simulink model "SecRwLtStBkReclnTrgtPosSelc"  (R2018b)
settings: Solver=FixedStepDiscrete  StartTime=0.0  StopTime=10.0  FixedStep=0.01  RelTol=1e-3
undefined symbols (not defined in the file): KeSMSw4SAcsMd21SecRwLtStBkReclnUpwdDnwdPos_Val, KeSMSw4SAcsMd21SecRwLtStBkReclnUpwdDnwdPosMax_Val, KeSMSw4SAcsMd21SecRwLtStBkReclnUpwdDnwdPosMin_Val, KeSMSw4SAcsMd22SecRwLtStBkReclnUpwdDnwdPos1_Val, KeSMSw4SAcsMd22SecRwLtStBkReclnUpwdDnwdPos1Max_Val, KeSMSw4SAcsMd22SecRwLtStBkReclnUpwdDnwdPos1Min_Val, KeSMSw4SAcsMd22SecRwLtStBkReclnUpwdDnwdPos2_Val, KeSMSw4SAcsMd22SecRwLtStBkReclnUpwdDnwdPos2Max_Val, KeSMSw4SAcsMd22SecRwLtStBkReclnUpwdDnwdPos2Min_Val, KeSMSw4SAcsMd25SecRwLtStBkReclnUpwdDnwdPos_Val, KeSMSw4SAcsMd25SecRwLtStBkReclnUpwdDnwdPosMax_Val, KeSMSw4SAcsMd25SecRwLtStBkReclnUpwdDnwdPosMin_Val, KeSMSw4SAcsMd26SecRwLtStBkReclnUpwdDnwdPos_Val, KeSMSw4SAcsMd26SecRwLtStBkReclnUpwdDnwdPosMax_Val, KeSMSw4SAcsMd26SecRwLtStBkReclnUpwdDnwdPosMin_Val, KeSMSw4sLyingMDSecRwLtStBkReclnUpwdDnwdPos_Val, KeSMSw4sLyingMDSecRwLtStBkReclnUpwdDnwdPosMax_Val, KeSMSw4sLyingMDSecRwLtStBkReclnUpwdDnwdPosMin_Val, KeSMSw4sRecoveryMDSecRwLtStBkReclnUpwdDnwdPos_Val, KeSMSw4sRecoveryMDSecRwLtStBkReclnUpwdDnwdPosMax_Val, KeSMSw4sRecoveryMDSecRwLtStBkReclnUpwdDnwdPosMin_Val, KeSMSw4sVIPMDSecRwLtStBkReclnUpwdDnwdPos_Val, KeSMSw4sVIPMDSecRwLtStBkReclnUpwdDnwdPosMax_Val, KeSMSw4sVIPMDSecRwLtStBkReclnUpwdDnwdPosMin_Val, KeSMSw6sAcsEntrySecRwLtStBkReclnUpwdDnwd1Pos_Val, KeSMSw6sAcsEntrySecRwLtStBkReclnUpwdDnwdPos1Max_Val, KeSMSw6sAcsEntrySecRwLtStBkReclnUpwdDnwdPos1Min_Val, KeSMSw6sAcsEntrySecRwLtStBkReclnUpwdDnwdPos_Val, KeSMSw6sAcsEntrySecRwLtStBkReclnUpwdDnwdPosMax_Val, KeSMSw6sAcsEntrySecRwLtStBkReclnUpwdDnwdPosMin_Val, KeSMSw6sAcsExtSecRwLtStBkReclnUpwdDnwdPos_Val, KeSMSw6sAcsExtSecRwLtStBkReclnUpwdDnwdPosMax_Val, KeSMSw6sAcsExtSecRwLtStBkReclnUpwdDnwdPosMin_Val, KeSMSw6sRecoveryMdSecRwLtStBkReclnUpwdDnwdPos_Val, KeSMSw6sRecoveryMdSecRwLtStBkReclnUpwdDnwdPosMax_Val, KeSMSw6sRecoveryMdSecRwLtStBkReclnUpwdDnwdPosMin_Val, KeSMSw6sVIPSecRwLtStBkReclnUpwdDnwdPos_Val, KeSMSw6sVIPSecRwLtStBkReclnUpwdDnwdPosMax_Val, KeSMSw6sVIPSecRwLtStBkReclnUpwdDnwdPosMin_Val, KeSMSwAcsEntrySecRwLtStBkReclnUpwdDnwdPos1_Val, KeSMSwAcsEntrySecRwLtStBkReclnUpwdDnwdPos1Max_Val, KeSMSwAcsEntrySecRwLtStBkReclnUpwdDnwdPos1Min_Val, KeSMSwAcsEntrySecRwLtStBkReclnUpwdDnwdPos_Val, KeSMSwAcsEntrySecRwLtStBkReclnUpwdDnwdPosMax_Val, KeSMSwAcsEntrySecRwLtStBkReclnUpwdDnwdPosMin_Val, KeSMSwAcsExtSecRwLtStBkReclnUpwdDnwdPos_Val, KeSMSwAcsExtSecRwLtStBkReclnUpwdDnwdPosMax_Val, KeSMSwAcsExtSecRwLtStBkReclnUpwdDnwdPosMin_Val, KeSMSwAcsMd32SecRwLtStBkReclnUpwdDnwdPos1_Val, KeSMSwAcsMd32SecRwLtStBkReclnUpwdDnwdPos1Max_Val, KeSMSwAcsMd32SecRwLtStBkReclnUpwdDnwdPos1Min_Val, KeSMSwAcsMd32SecRwLtStBkReclnUpwdDnwdPos_Val, KeSMSwAcsMd32SecRwLtStBkReclnUpwdDnwdPosMax_Val, KeSMSwAcsMd32SecRwLtStBkReclnUpwdDnwdPosMin_Val, KeSMSwAcsMd8SecRwLtStBkReclnUpwdDnwdPos_Val, KeSMSwAcsMd8SecRwLtStBkReclnUpwdDnwdPosMax_Val, KeSMSwAcsMd8SecRwLtStBkReclnUpwdDnwdPosMin_Val, KeSMSwRecoveryMdSecRwLtStBkReclnUpwdDnwdPos_Val, KeSMSwRecoveryMdSecRwLtStBkReclnUpwdDnwdPosMax_Val, KeSMSwRecoveryMdSecRwLtStBkReclnUpwdDnwdPosMin_Val ... (+3)
libraries: TrgtPosSelcLib x13, StIsPosChkLib x1, simulink x1
(part 1 of 2)
settings Model: Creator=sn2xws  LastModifiedBy=sn2xws
settings Model: ModifiedHistory=|
  | 2023.8.1 V2.0.0 CR421790 增加模式21-26
  | 2023.11.7 V2.3.0 bug 554442 md22 标定分为两套
  | 2024.5.7 557 eze模式变更
  | 2024.7.8 V3.0.1 557模式流程V1.9
  | 2024.8.17 V3.0.2 MD1靠背阶段1，2的选择逻辑变更
  | 2024.8.20 V3.0.3 Md32 目标位置改用Cush位置选择
settings DataIOCC: SaveFormat=StructureWithTime
settings OptimizationCC: DefaultParameterBehavior=Inlined  EnhancedBackFolding=on  PassReuseOutputArgsAs=Individual arguments  ZeroExternalMemoryAtStartup=off  ZeroInternalMemoryAtStartup=off  OptimizeBlockOrder=speed  DifferentSizesBufferReuse=on  OptimizationCustomize=off
settings DebuggingCC: ParameterTunabilityLossMsg=error
settings SFSimCC: MATLABDynamicMemAlloc=off
settings RTWCC: SystemTargetFile=autosar.tlc  GenCodeOnly=on  TemplateMakefile=ert_default_tmf  Description=AUTOSAR  GenerateReport=on  IncludeHyperlinkInReport=on  LaunchReport=on  GenerateTraceInfo=on  GenerateTraceReport=on  GenerateTraceReportSl=on  GenerateTraceReportSf=on  GenerateTraceReportEml=on  GenerateCodeMetricsReport=on
settings CodeAppCC: ForceParamTrailComments=on  IgnoreCustomStorageClasses=off  OperatorAnnotations=on  SimulinkDataObjDesc=on  SFDataObjDesc=on  InsertBlockDesc=on
settings STFCustomTargetCC: TargetLangStandard=C99 (ISO)  MultiwordLength=256  ParMdlRefBuildCompliant=on  CompOptLevelCompliant=on  IncludeMdlTerminateFcn=off  CombineOutputUpdateFcns=on  SuppressErrorStatus=on  ERTCustomFileBanners=on  SupportNonFinite=off  SupportComplex=off  SupportContinuousTime=off  SupportNonInlinedSFcns=off  RemoveResetFunc=on  MATLABClassNameForMDSCustomization=Simulink.SoftwareTarget.ERTCustomization  AutosarCompliant=on  UseToolchainInfoCompliant=on  LookupTableObjectStructAxisOrder=2,1,3,4,...  LUTObjectStructOrderEvenSpacing=Size,Table,Breakpoints  SystemTargetFile=autosar.tlc
settings ERTTargetCC: TargetLangStandard=C99 (ISO)  ConcurrentExecutionCompliant=off  IncludeMdlTerminateFcn=off  SuppressErrorStatus=on  SupportNonFinite=off  SupportComplex=off  ModelStepFunctionPrototypeControlCompliant=off  CPPClassGenCompliant=off  AutosarCompliant=on  LookupTableObjectStructAxisOrder=2,1,3,4,...  LUTObjectStructOrderEvenSpacing=Size,Table,Breakpoints  InlinedParameterPlacement=NonHierarchical  ERTCustomFileTemplate=example_file_process.tlc  ERTFilePackagingFormat=Compact

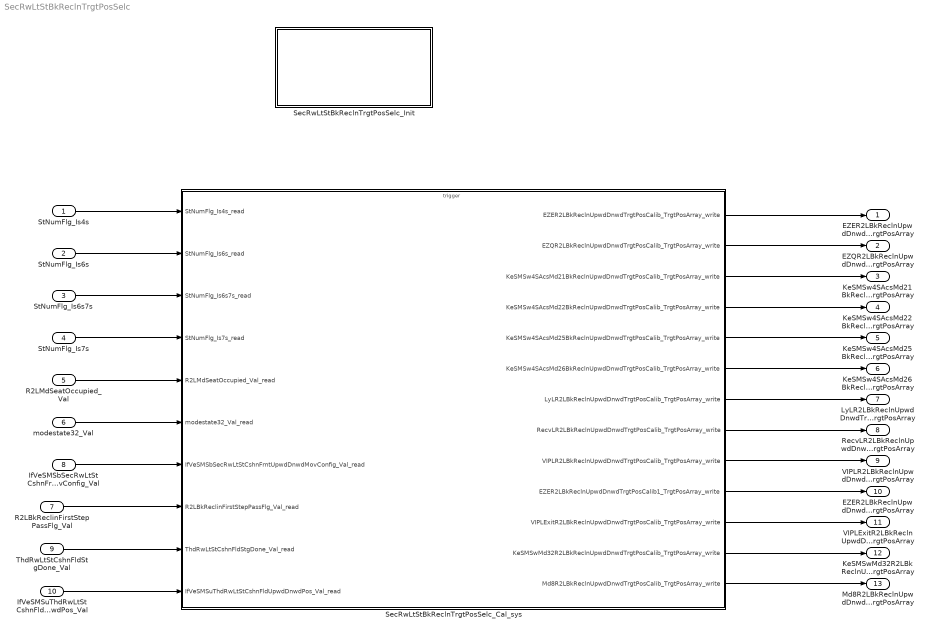
== system SecRwLtStBkReclnTrgtPosSelc ==
  StNumFlg_Is4s : Inport  OutDataTypeStr=boolean  PortDimensions=1
  StNumFlg_Is6s : Inport  Port=2  OutDataTypeStr=boolean  PortDimensions=1
  StNumFlg_Is6s7s : Inport  Port=3  OutDataTypeStr=boolean  PortDimensions=1
  StNumFlg_Is7s : Inport  Port=4  OutDataTypeStr=boolean  PortDimensions=1
  R2LMdSeatOccupied_Val : Inport  Port=5  OutDataTypeStr=boolean  PortDimensions=1
  modestate32_Val : Inport  Port=6  OutDataTypeStr=uint32  PortDimensions=1
  R2LBkReclinFirstStepPassFlg_Val : Inport  Port=7  OutDataTypeStr=boolean  PortDimensions=1
  IfVeSMSbSecRwLtStCshnFrntUpwdDnwdMovConfig_Val : Inport  Port=8  OutDataTypeStr=boolean  PortDimensions=1
  ThdRwLtStCshnFldStgDone_Val : Inport  Port=9  OutDataTypeStr=boolean  PortDimensions=1
  IfVeSMSuThdRwLtStCshnFldUpwdDnwdPos_Val : Inport  Port=10  OutDataTypeStr=uint16  PortDimensions=1
  SecRwLtStBkReclnTrgtPosSelc_Cal_sys : Subsystem
  SecRwLtStBkReclnTrgtPosSelc_Init : Subsystem
  EZER2LBkReclnUpwdDnwdTrgtPosCalib_TrgtPosArray : Outport  Description=|  OutDataTypeStr=uint16  PortDimensions=3
      | 0:Pos
      | 1:Max
      | 2:Min
  EZQR2LBkReclnUpwdDnwdTrgtPosCalib_TrgtPosArray : Outport  Description=|  Port=2  OutDataTypeStr=uint16  PortDimensions=3
      | 0:Pos
      | 1:Max
      | 2:Min
  KeSMSw4SAcsMd21BkReclnUpwdDnwdTrgtPosCalib_TrgtPosArray : Outport  Description=|  Port=3  OutDataTypeStr=uint16  PortDimensions=3
      | 0:Pos
      | 1:Max
      | 2:Min
  KeSMSw4SAcsMd22BkReclnUpwdDnwdTrgtPosCalib_TrgtPosArray : Outport  Description=|  Port=4  OutDataTypeStr=uint16  PortDimensions=3
      | 0:Pos
      | 1:Max
      | 2:Min
  KeSMSw4SAcsMd25BkReclnUpwdDnwdTrgtPosCalib_TrgtPosArray : Outport  Description=|  Port=5  OutDataTypeStr=uint16  PortDimensions=3
      | 0:Pos
      | 1:Max
      | 2:Min
  KeSMSw4SAcsMd26BkReclnUpwdDnwdTrgtPosCalib_TrgtPosArray : Outport  Description=|  Port=6  OutDataTypeStr=uint16  PortDimensions=3
      | 0:Pos
      | 1:Max
      | 2:Min
  LyLR2LBkReclnUpwdDnwdTrgtPosCalib_TrgtPosArray : Outport  Description=|  Port=7  OutDataTypeStr=uint16  PortDimensions=3
      | 0:Pos
      | 1:Max
      | 2:Min
  RecvLR2LBkReclnUpwdDnwdTrgtPosCalib_TrgtPosArray : Outport  Description=|  Port=8  OutDataTypeStr=uint16  PortDimensions=3
      | 0:Pos
      | 1:Max
      | 2:Min
  VIPLR2LBkReclnUpwdDnwdTrgtPosCalib_TrgtPosArray : Outport  Description=|  Port=9  OutDataTypeStr=uint16  PortDimensions=3
      | 0:Pos
      | 1:Max
      | 2:Min
  EZER2LBkReclnUpwdDnwdTrgtPosCalib1_TrgtPosArray : Outport  Description=|  Port=10  OutDataTypeStr=uint16  PortDimensions=3
      | 0:Pos
      | 1:Max
      | 2:Min
  VIPLExitR2LBkReclnUpwdDnwdTrgtPosCalib_TrgtPosArray : Outport  Description=|  Port=11  OutDataTypeStr=uint16  PortDimensions=3
      | 0:Pos
      | 1:Max
      | 2:Min
  KeSMSwMd32R2LBkReclnUpwdDnwdTrgtPosCalib_TrgtPosArray : Outport  Description=|  Port=12  OutDataTypeStr=uint16  PortDimensions=3
      | 0:Pos
      | 1:Max
      | 2:Min
  Md8R2LBkReclnUpwdDnwdTrgtPosCalib_TrgtPosArray : Outport  Description=|  Port=13  OutDataTypeStr=uint16  PortDimensions=3
      | 0:Pos
      | 1:Max
      | 2:Min
  wires:
  StNumFlg_Is4s/1 -> SecRwLtStBkReclnTrgtPosSelc_Cal_sys/1(StNumFlg_Is4s_read)
  StNumFlg_Is6s/1 -> SecRwLtStBkReclnTrgtPosSelc_Cal_sys/2(StNumFlg_Is6s_read)
  StNumFlg_Is6s7s/1 -> SecRwLtStBkReclnTrgtPosSelc_Cal_sys/3(StNumFlg_Is6s7s_read)
  StNumFlg_Is7s/1 -> SecRwLtStBkReclnTrgtPosSelc_Cal_sys/4(StNumFlg_Is7s_read)
  SecRwLtStBkReclnTrgtPosSelc_Cal_sys/1(EZER2LBkReclnUpwdDnwdTrgtPosCalib_TrgtPosArray_write) -> EZER2LBkReclnUpwdDnwdTrgtPosCalib_TrgtPosArray/1
  SecRwLtStBkReclnTrgtPosSelc_Cal_sys/2(EZQR2LBkReclnUpwdDnwdTrgtPosCalib_TrgtPosArray_write) -> EZQR2LBkReclnUpwdDnwdTrgtPosCalib_TrgtPosArray/1
  SecRwLtStBkReclnTrgtPosSelc_Cal_sys/3(KeSMSw4SAcsMd21BkReclnUpwdDnwdTrgtPosCalib_TrgtPosArray_write) -> KeSMSw4SAcsMd21BkReclnUpwdDnwdTrgtPosCalib_TrgtPosArray/1
  SecRwLtStBkReclnTrgtPosSelc_Cal_sys/4(KeSMSw4SAcsMd22BkReclnUpwdDnwdTrgtPosCalib_TrgtPosArray_write) -> KeSMSw4SAcsMd22BkReclnUpwdDnwdTrgtPosCalib_TrgtPosArray/1
  SecRwLtStBkReclnTrgtPosSelc_Cal_sys/5(KeSMSw4SAcsMd25BkReclnUpwdDnwdTrgtPosCalib_TrgtPosArray_write) -> KeSMSw4SAcsMd25BkReclnUpwdDnwdTrgtPosCalib_TrgtPosArray/1
  SecRwLtStBkReclnTrgtPosSelc_Cal_sys/6(KeSMSw4SAcsMd26BkReclnUpwdDnwdTrgtPosCalib_TrgtPosArray_write) -> KeSMSw4SAcsMd26BkReclnUpwdDnwdTrgtPosCalib_TrgtPosArray/1
  SecRwLtStBkReclnTrgtPosSelc_Cal_sys/7(LyLR2LBkReclnUpwdDnwdTrgtPosCalib_TrgtPosArray_write) -> LyLR2LBkReclnUpwdDnwdTrgtPosCalib_TrgtPosArray/1
  SecRwLtStBkReclnTrgtPosSelc_Cal_sys/8(RecvLR2LBkReclnUpwdDnwdTrgtPosCalib_TrgtPosArray_write) -> RecvLR2LBkReclnUpwdDnwdTrgtPosCalib_TrgtPosArray/1
  SecRwLtStBkReclnTrgtPosSelc_Cal_sys/9(VIPLR2LBkReclnUpwdDnwdTrgtPosCalib_TrgtPosArray_write) -> VIPLR2LBkReclnUpwdDnwdTrgtPosCalib_TrgtPosArray/1
  R2LMdSeatOccupied_Val/1 -> SecRwLtStBkReclnTrgtPosSelc_Cal_sys/5(R2LMdSeatOccupied_Val_read)
  SecRwLtStBkReclnTrgtPosSelc_Cal_sys/10(EZER2LBkReclnUpwdDnwdTrgtPosCalib1_TrgtPosArray_write) -> EZER2LBkReclnUpwdDnwdTrgtPosCalib1_TrgtPosArray/1
  modestate32_Val/1 -> SecRwLtStBkReclnTrgtPosSelc_Cal_sys/6(modestate32_Val_read)
  R2LBkReclinFirstStepPassFlg_Val/1 -> SecRwLtStBkReclnTrgtPosSelc_Cal_sys/8(R2LBkReclinFirstStepPassFlg_Val_read)
  IfVeSMSbSecRwLtStCshnFrntUpwdDnwdMovConfig_Val/1 -> SecRwLtStBkReclnTrgtPosSelc_Cal_sys/7(IfVeSMSbSecRwLtStCshnFrntUpwdDnwdMovConfig_Val_read)
  SecRwLtStBkReclnTrgtPosSelc_Cal_sys/11(VIPLExitR2LBkReclnUpwdDnwdTrgtPosCalib_TrgtPosArray_write) -> VIPLExitR2LBkReclnUpwdDnwdTrgtPosCalib_TrgtPosArray/1
  ThdRwLtStCshnFldStgDone_Val/1 -> SecRwLtStBkReclnTrgtPosSelc_Cal_sys/9(ThdRwLtStCshnFldStgDone_Val_read)
  SecRwLtStBkReclnTrgtPosSelc_Cal_sys/12(KeSMSwMd32R2LBkReclnUpwdDnwdTrgtPosCalib_TrgtPosArray_write) -> KeSMSwMd32R2LBkReclnUpwdDnwdTrgtPosCalib_TrgtPosArray/1
  SecRwLtStBkReclnTrgtPosSelc_Cal_sys/13(Md8R2LBkReclnUpwdDnwdTrgtPosCalib_TrgtPosArray_write) -> Md8R2LBkReclnUpwdDnwdTrgtPosCalib_TrgtPosArray/1
  IfVeSMSuThdRwLtStCshnFldUpwdDnwdPos_Val/1 -> SecRwLtStBkReclnTrgtPosSelc_Cal_sys/10(IfVeSMSuThdRwLtStCshnFldUpwdDnwdPos_Val_read)

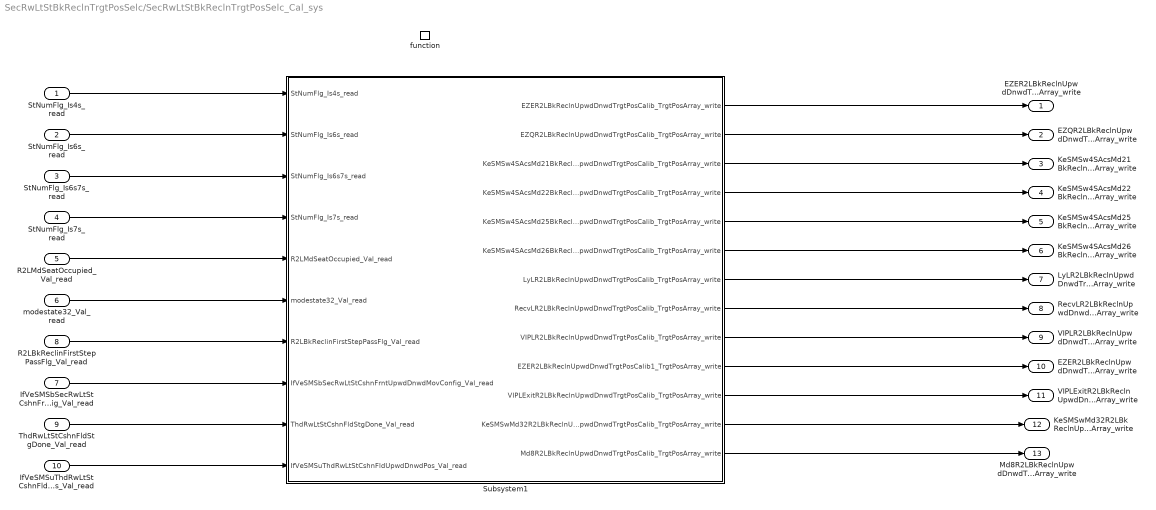
== system SecRwLtStBkReclnTrgtPosSelc/SecRwLtStBkReclnTrgtPosSelc_Cal_sys ==
  StNumFlg_Is4s_read : Inport
  StNumFlg_Is6s_read : Inport  Port=2
  StNumFlg_Is6s7s_read : Inport  Port=3
  StNumFlg_Is7s_read : Inport  Port=4
  R2LMdSeatOccupied_Val_read : Inport  Port=5
  modestate32_Val_read : Inport  Port=6
  IfVeSMSbSecRwLtStCshnFrntUpwdDnwdMovConfig_Val_read : Inport  Port=7
  R2LBkReclinFirstStepPassFlg_Val_read : Inport  Port=8
  ThdRwLtStCshnFldStgDone_Val_read : Inport  Port=9
  IfVeSMSuThdRwLtStCshnFldUpwdDnwdPos_Val_read : Inport  Port=10
  function : TriggerPort  TriggerType=function-call  IsSimulinkFunction=on  FunctionName=SecRwLtStBkReclnTrgtPosSelc_Cal  VariantControl=(inherit)
  Subsystem1 : Subsystem
  EZER2LBkReclnUpwdDnwdTrgtPosCalib_TrgtPosArray_write : Outport
      settings: EnsureOutportIsVirtual=on
  EZQR2LBkReclnUpwdDnwdTrgtPosCalib_TrgtPosArray_write : Outport  Port=2
      settings: EnsureOutportIsVirtual=on
  KeSMSw4SAcsMd21BkReclnUpwdDnwdTrgtPosCalib_TrgtPosArray_write : Outport  Port=3
      settings: EnsureOutportIsVirtual=on
  KeSMSw4SAcsMd22BkReclnUpwdDnwdTrgtPosCalib_TrgtPosArray_write : Outport  Port=4
      settings: EnsureOutportIsVirtual=on
  KeSMSw4SAcsMd25BkReclnUpwdDnwdTrgtPosCalib_TrgtPosArray_write : Outport  Port=5
      settings: EnsureOutportIsVirtual=on
  KeSMSw4SAcsMd26BkReclnUpwdDnwdTrgtPosCalib_TrgtPosArray_write : Outport  Port=6
      settings: EnsureOutportIsVirtual=on
  LyLR2LBkReclnUpwdDnwdTrgtPosCalib_TrgtPosArray_write : Outport  Port=7
      settings: EnsureOutportIsVirtual=on
  RecvLR2LBkReclnUpwdDnwdTrgtPosCalib_TrgtPosArray_write : Outport  Port=8
      settings: EnsureOutportIsVirtual=on
  VIPLR2LBkReclnUpwdDnwdTrgtPosCalib_TrgtPosArray_write : Outport  Port=9
      settings: EnsureOutportIsVirtual=on
  EZER2LBkReclnUpwdDnwdTrgtPosCalib1_TrgtPosArray_write : Outport  Port=10
      settings: EnsureOutportIsVirtual=on
  VIPLExitR2LBkReclnUpwdDnwdTrgtPosCalib_TrgtPosArray_write : Outport  Port=11
      settings: EnsureOutportIsVirtual=on
  KeSMSwMd32R2LBkReclnUpwdDnwdTrgtPosCalib_TrgtPosArray_write : Outport  Port=12
      settings: EnsureOutportIsVirtual=on
  Md8R2LBkReclnUpwdDnwdTrgtPosCalib_TrgtPosArray_write : Outport  Port=13
      settings: EnsureOutportIsVirtual=on
  wires:
  Subsystem1/6(KeSMSw4SAcsMd26BkReclnUpwdDnwdTrgtPosCalib_TrgtPosArray_write) -> KeSMSw4SAcsMd26BkReclnUpwdDnwdTrgtPosCalib_TrgtPosArray_write/1
  Subsystem1/7(LyLR2LBkReclnUpwdDnwdTrgtPosCalib_TrgtPosArray_write) -> LyLR2LBkReclnUpwdDnwdTrgtPosCalib_TrgtPosArray_write/1
  Subsystem1/8(RecvLR2LBkReclnUpwdDnwdTrgtPosCalib_TrgtPosArray_write) -> RecvLR2LBkReclnUpwdDnwdTrgtPosCalib_TrgtPosArray_write/1
  Subsystem1/4(KeSMSw4SAcsMd22BkReclnUpwdDnwdTrgtPosCalib_TrgtPosArray_write) -> KeSMSw4SAcsMd22BkReclnUpwdDnwdTrgtPosCalib_TrgtPosArray_write/1
  Subsystem1/5(KeSMSw4SAcsMd25BkReclnUpwdDnwdTrgtPosCalib_TrgtPosArray_write) -> KeSMSw4SAcsMd25BkReclnUpwdDnwdTrgtPosCalib_TrgtPosArray_write/1
  Subsystem1/9(VIPLR2LBkReclnUpwdDnwdTrgtPosCalib_TrgtPosArray_write) -> VIPLR2LBkReclnUpwdDnwdTrgtPosCalib_TrgtPosArray_write/1
  Subsystem1/1(EZER2LBkReclnUpwdDnwdTrgtPosCalib_TrgtPosArray_write) -> EZER2LBkReclnUpwdDnwdTrgtPosCalib_TrgtPosArray_write/1
  Subsystem1/2(EZQR2LBkReclnUpwdDnwdTrgtPosCalib_TrgtPosArray_write) -> EZQR2LBkReclnUpwdDnwdTrgtPosCalib_TrgtPosArray_write/1
  Subsystem1/3(KeSMSw4SAcsMd21BkReclnUpwdDnwdTrgtPosCalib_TrgtPosArray_write) -> KeSMSw4SAcsMd21BkReclnUpwdDnwdTrgtPosCalib_TrgtPosArray_write/1
  StNumFlg_Is4s_read/1 -> Subsystem1/1(StNumFlg_Is4s_read)
  StNumFlg_Is6s_read/1 -> Subsystem1/2(StNumFlg_Is6s_read)
  StNumFlg_Is6s7s_read/1 -> Subsystem1/3(StNumFlg_Is6s7s_read)
  StNumFlg_Is7s_read/1 -> Subsystem1/4(StNumFlg_Is7s_read)
  R2LMdSeatOccupied_Val_read/1 -> Subsystem1/5(R2LMdSeatOccupied_Val_read)
  Subsystem1/10(EZER2LBkReclnUpwdDnwdTrgtPosCalib1_TrgtPosArray_write) -> EZER2LBkReclnUpwdDnwdTrgtPosCalib1_TrgtPosArray_write/1
  modestate32_Val_read/1 -> Subsystem1/6(modestate32_Val_read)
  IfVeSMSbSecRwLtStCshnFrntUpwdDnwdMovConfig_Val_read/1 -> Subsystem1/8(IfVeSMSbSecRwLtStCshnFrntUpwdDnwdMovConfig_Val_read)
  Subsystem1/11(VIPLExitR2LBkReclnUpwdDnwdTrgtPosCalib_TrgtPosArray_write) -> VIPLExitR2LBkReclnUpwdDnwdTrgtPosCalib_TrgtPosArray_write/1
  Subsystem1/12(KeSMSwMd32R2LBkReclnUpwdDnwdTrgtPosCalib_TrgtPosArray_write) -> KeSMSwMd32R2LBkReclnUpwdDnwdTrgtPosCalib_TrgtPosArray_write/1
  Subsystem1/13(Md8R2LBkReclnUpwdDnwdTrgtPosCalib_TrgtPosArray_write) -> Md8R2LBkReclnUpwdDnwdTrgtPosCalib_TrgtPosArray_write/1
  R2LBkReclinFirstStepPassFlg_Val_read/1 -> Subsystem1/7(R2LBkReclinFirstStepPassFlg_Val_read)
  ThdRwLtStCshnFldStgDone_Val_read/1 -> Subsystem1/9(ThdRwLtStCshnFldStgDone_Val_read)
  IfVeSMSuThdRwLtStCshnFldUpwdDnwdPos_Val_read/1 -> Subsystem1/10(IfVeSMSuThdRwLtStCshnFldUpwdDnwdPos_Val_read)

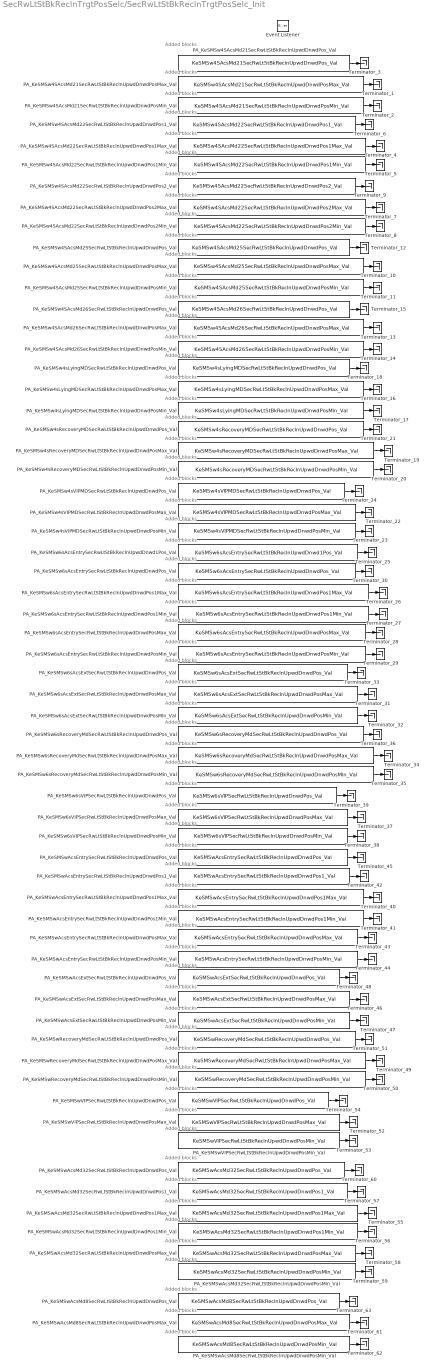
== system SecRwLtStBkReclnTrgtPosSelc/SecRwLtStBkReclnTrgtPosSelc_Init ==
  note: Added blocks
  note: Added blocks
  note: Added blocks
  note: Added blocks
  note: Added blocks
  note: Added blocks
  note: Added blocks
  note: Added blocks
  note: Added blocks
  note: Added blocks
  note: Added blocks
  note: Added blocks
  note: Added blocks
  note: Added blocks
  note: Added blocks
  note: Added blocks
  note: Added blocks
  note: Added blocks
  note: Added blocks
  note: Added blocks
  note: Added blocks
  note: Added blocks
  note: Added blocks
  note: Added blocks
  note: Added blocks
  note: Added blocks
  note: Added blocks
  note: Added blocks
  note: Added blocks
  note: Added blocks
  note: Added blocks
  note: Added blocks
  note: Added blocks
  note: Added blocks
  note: Added blocks
  note: Added blocks
  note: Added blocks
  note: Added blocks
  note: Added blocks
  note: Added blocks
  note: Added blocks
  note: Added blocks
  note: Added blocks
  note: Added blocks
  note: Added blocks
  note: Added blocks
  note: Added blocks
  note: Added blocks
  note: Added blocks
  note: Added blocks
  note: Added blocks
  note: Added blocks
  note: Added blocks
  note: Added blocks
  note: Added blocks
  note: Added blocks
  note: Added blocks
  note: Added blocks
  note: Added blocks
  note: Added blocks
  note: Added blocks
  note: Added blocks
  note: Added blocks
  Event Listener : EventListener  EventName=reset
  PA_KeSMSw4SAcsMd21SecRwLtStBkReclnUpwdDnwdPosMax_Val : Constant  Value=KeSMSw4SAcsMd21SecRwLtStBkReclnUpwdDnwdPosMax_Val
  PA_KeSMSw4SAcsMd21SecRwLtStBkReclnUpwdDnwdPosMin_Val : Constant  Value=KeSMSw4SAcsMd21SecRwLtStBkReclnUpwdDnwdPosMin_Val
  PA_KeSMSw4SAcsMd21SecRwLtStBkReclnUpwdDnwdPos_Val : Constant  Value=KeSMSw4SAcsMd21SecRwLtStBkReclnUpwdDnwdPos_Val
  PA_KeSMSw4SAcsMd22SecRwLtStBkReclnUpwdDnwdPos1Max_Val : Constant  Value=KeSMSw4SAcsMd22SecRwLtStBkReclnUpwdDnwdPos1Max_Val
  PA_KeSMSw4SAcsMd22SecRwLtStBkReclnUpwdDnwdPos1Min_Val : Constant  Value=KeSMSw4SAcsMd22SecRwLtStBkReclnUpwdDnwdPos1Min_Val
  PA_KeSMSw4SAcsMd22SecRwLtStBkReclnUpwdDnwdPos1_Val : Constant  Value=KeSMSw4SAcsMd22SecRwLtStBkReclnUpwdDnwdPos1_Val
  PA_KeSMSw4SAcsMd22SecRwLtStBkReclnUpwdDnwdPos2Max_Val : Constant  Value=KeSMSw4SAcsMd22SecRwLtStBkReclnUpwdDnwdPos2Max_Val
  PA_KeSMSw4SAcsMd22SecRwLtStBkReclnUpwdDnwdPos2Min_Val : Constant  Value=KeSMSw4SAcsMd22SecRwLtStBkReclnUpwdDnwdPos2Min_Val
  PA_KeSMSw4SAcsMd22SecRwLtStBkReclnUpwdDnwdPos2_Val : Constant  Value=KeSMSw4SAcsMd22SecRwLtStBkReclnUpwdDnwdPos2_Val
  PA_KeSMSw4SAcsMd25SecRwLtStBkReclnUpwdDnwdPosMax_Val : Constant  Value=KeSMSw4SAcsMd25SecRwLtStBkReclnUpwdDnwdPosMax_Val
  PA_KeSMSw4SAcsMd25SecRwLtStBkReclnUpwdDnwdPosMin_Val : Constant  Value=KeSMSw4SAcsMd25SecRwLtStBkReclnUpwdDnwdPosMin_Val
  PA_KeSMSw4SAcsMd25SecRwLtStBkReclnUpwdDnwdPos_Val : Constant  Value=KeSMSw4SAcsMd25SecRwLtStBkReclnUpwdDnwdPos_Val
  PA_KeSMSw4SAcsMd26SecRwLtStBkReclnUpwdDnwdPosMax_Val : Constant  Value=KeSMSw4SAcsMd26SecRwLtStBkReclnUpwdDnwdPosMax_Val
  PA_KeSMSw4SAcsMd26SecRwLtStBkReclnUpwdDnwdPosMin_Val : Constant  Value=KeSMSw4SAcsMd26SecRwLtStBkReclnUpwdDnwdPosMin_Val
  PA_KeSMSw4SAcsMd26SecRwLtStBkReclnUpwdDnwdPos_Val : Constant  Value=KeSMSw4SAcsMd26SecRwLtStBkReclnUpwdDnwdPos_Val
  PA_KeSMSw4sLyingMDSecRwLtStBkReclnUpwdDnwdPosMax_Val : Constant  Value=KeSMSw4sLyingMDSecRwLtStBkReclnUpwdDnwdPosMax_Val
  PA_KeSMSw4sLyingMDSecRwLtStBkReclnUpwdDnwdPosMin_Val : Constant  Value=KeSMSw4sLyingMDSecRwLtStBkReclnUpwdDnwdPosMin_Val
  PA_KeSMSw4sLyingMDSecRwLtStBkReclnUpwdDnwdPos_Val : Constant  Value=KeSMSw4sLyingMDSecRwLtStBkReclnUpwdDnwdPos_Val
  PA_KeSMSw4sRecoveryMDSecRwLtStBkReclnUpwdDnwdPosMax_Val : Constant  Value=KeSMSw4sRecoveryMDSecRwLtStBkReclnUpwdDnwdPosMax_Val
  PA_KeSMSw4sRecoveryMDSecRwLtStBkReclnUpwdDnwdPosMin_Val : Constant  Value=KeSMSw4sRecoveryMDSecRwLtStBkReclnUpwdDnwdPosMin_Val
  PA_KeSMSw4sRecoveryMDSecRwLtStBkReclnUpwdDnwdPos_Val : Constant  Value=KeSMSw4sRecoveryMDSecRwLtStBkReclnUpwdDnwdPos_Val
  PA_KeSMSw4sVIPMDSecRwLtStBkReclnUpwdDnwdPosMax_Val : Constant  Value=KeSMSw4sVIPMDSecRwLtStBkReclnUpwdDnwdPosMax_Val
  PA_KeSMSw4sVIPMDSecRwLtStBkReclnUpwdDnwdPosMin_Val : Constant  Value=KeSMSw4sVIPMDSecRwLtStBkReclnUpwdDnwdPosMin_Val
  PA_KeSMSw4sVIPMDSecRwLtStBkReclnUpwdDnwdPos_Val : Constant  Value=KeSMSw4sVIPMDSecRwLtStBkReclnUpwdDnwdPos_Val
  PA_KeSMSw6sAcsEntrySecRwLtStBkReclnUpwdDnwd1Pos_Val : Constant  Value=KeSMSw6sAcsEntrySecRwLtStBkReclnUpwdDnwd1Pos_Val
  PA_KeSMSw6sAcsEntrySecRwLtStBkReclnUpwdDnwdPos1Max_Val : Constant  Value=KeSMSw6sAcsEntrySecRwLtStBkReclnUpwdDnwdPos1Max_Val
  PA_KeSMSw6sAcsEntrySecRwLtStBkReclnUpwdDnwdPos1Min_Val : Constant  Value=KeSMSw6sAcsEntrySecRwLtStBkReclnUpwdDnwdPos1Min_Val
  PA_KeSMSw6sAcsEntrySecRwLtStBkReclnUpwdDnwdPosMax_Val : Constant  Value=KeSMSw6sAcsEntrySecRwLtStBkReclnUpwdDnwdPosMax_Val
  PA_KeSMSw6sAcsEntrySecRwLtStBkReclnUpwdDnwdPosMin_Val : Constant  Value=KeSMSw6sAcsEntrySecRwLtStBkReclnUpwdDnwdPosMin_Val
  PA_KeSMSw6sAcsEntrySecRwLtStBkReclnUpwdDnwdPos_Val : Constant  Value=KeSMSw6sAcsEntrySecRwLtStBkReclnUpwdDnwdPos_Val
  PA_KeSMSw6sAcsExtSecRwLtStBkReclnUpwdDnwdPosMax_Val : Constant  Value=KeSMSw6sAcsExtSecRwLtStBkReclnUpwdDnwdPosMax_Val
  PA_KeSMSw6sAcsExtSecRwLtStBkReclnUpwdDnwdPosMin_Val : Constant  Value=KeSMSw6sAcsExtSecRwLtStBkReclnUpwdDnwdPosMin_Val
  PA_KeSMSw6sAcsExtSecRwLtStBkReclnUpwdDnwdPos_Val : Constant  Value=KeSMSw6sAcsExtSecRwLtStBkReclnUpwdDnwdPos_Val
  PA_KeSMSw6sRecoveryMdSecRwLtStBkReclnUpwdDnwdPosMax_Val : Constant  Value=KeSMSw6sRecoveryMdSecRwLtStBkReclnUpwdDnwdPosMax_Val
  PA_KeSMSw6sRecoveryMdSecRwLtStBkReclnUpwdDnwdPosMin_Val : Constant  Value=KeSMSw6sRecoveryMdSecRwLtStBkReclnUpwdDnwdPosMin_Val
  PA_KeSMSw6sRecoveryMdSecRwLtStBkReclnUpwdDnwdPos_Val : Constant  Value=KeSMSw6sRecoveryMdSecRwLtStBkReclnUpwdDnwdPos_Val
  PA_KeSMSw6sVIPSecRwLtStBkReclnUpwdDnwdPosMax_Val : Constant  Value=KeSMSw6sVIPSecRwLtStBkReclnUpwdDnwdPosMax_Val
  PA_KeSMSw6sVIPSecRwLtStBkReclnUpwdDnwdPosMin_Val : Constant  Value=KeSMSw6sVIPSecRwLtStBkReclnUpwdDnwdPosMin_Val
  PA_KeSMSw6sVIPSecRwLtStBkReclnUpwdDnwdPos_Val : Constant  Value=KeSMSw6sVIPSecRwLtStBkReclnUpwdDnwdPos_Val
  PA_KeSMSwAcsEntrySecRwLtStBkReclnUpwdDnwdPos1Max_Val : Constant  Value=KeSMSwAcsEntrySecRwLtStBkReclnUpwdDnwdPos1Max_Val
  PA_KeSMSwAcsEntrySecRwLtStBkReclnUpwdDnwdPos1Min_Val : Constant  Value=KeSMSwAcsEntrySecRwLtStBkReclnUpwdDnwdPos1Min_Val
  PA_KeSMSwAcsEntrySecRwLtStBkReclnUpwdDnwdPos1_Val : Constant  Value=KeSMSwAcsEntrySecRwLtStBkReclnUpwdDnwdPos1_Val
  PA_KeSMSwAcsEntrySecRwLtStBkReclnUpwdDnwdPosMax_Val : Constant  Value=KeSMSwAcsEntrySecRwLtStBkReclnUpwdDnwdPosMax_Val
  PA_KeSMSwAcsEntrySecRwLtStBkReclnUpwdDnwdPosMin_Val : Constant  Value=KeSMSwAcsEntrySecRwLtStBkReclnUpwdDnwdPosMin_Val
  PA_KeSMSwAcsEntrySecRwLtStBkReclnUpwdDnwdPos_Val : Constant  Value=KeSMSwAcsEntrySecRwLtStBkReclnUpwdDnwdPos_Val
  PA_KeSMSwAcsExtSecRwLtStBkReclnUpwdDnwdPosMax_Val : Constant  Value=KeSMSwAcsExtSecRwLtStBkReclnUpwdDnwdPosMax_Val
  PA_KeSMSwAcsExtSecRwLtStBkReclnUpwdDnwdPosMin_Val : Constant  Value=KeSMSwAcsExtSecRwLtStBkReclnUpwdDnwdPosMin_Val
  PA_KeSMSwAcsExtSecRwLtStBkReclnUpwdDnwdPos_Val : Constant  Value=KeSMSwAcsExtSecRwLtStBkReclnUpwdDnwdPos_Val
  PA_KeSMSwAcsMd32SecRwLtStBkReclnUpwdDnwdPos1Max_Val : Constant  Value=KeSMSwAcsMd32SecRwLtStBkReclnUpwdDnwdPos1Max_Val
  PA_KeSMSwAcsMd32SecRwLtStBkReclnUpwdDnwdPos1Min_Val : Constant  Value=KeSMSwAcsMd32SecRwLtStBkReclnUpwdDnwdPos1Min_Val
  PA_KeSMSwAcsMd32SecRwLtStBkReclnUpwdDnwdPos1_Val : Constant  Value=KeSMSwAcsMd32SecRwLtStBkReclnUpwdDnwdPos1_Val
  PA_KeSMSwAcsMd32SecRwLtStBkReclnUpwdDnwdPosMax_Val : Constant  Value=KeSMSwAcsMd32SecRwLtStBkReclnUpwdDnwdPosMax_Val
  PA_KeSMSwAcsMd32SecRwLtStBkReclnUpwdDnwdPosMin_Val : Constant  Value=KeSMSwAcsMd32SecRwLtStBkReclnUpwdDnwdPosMin_Val
  PA_KeSMSwAcsMd32SecRwLtStBkReclnUpwdDnwdPos_Val : Constant  Value=KeSMSwAcsMd32SecRwLtStBkReclnUpwdDnwdPos_Val
  PA_KeSMSwAcsMd8SecRwLtStBkReclnUpwdDnwdPosMax_Val : Constant  Value=KeSMSwAcsMd8SecRwLtStBkReclnUpwdDnwdPosMax_Val
  PA_KeSMSwAcsMd8SecRwLtStBkReclnUpwdDnwdPosMin_Val : Constant  Value=KeSMSwAcsMd8SecRwLtStBkReclnUpwdDnwdPosMin_Val
  PA_KeSMSwAcsMd8SecRwLtStBkReclnUpwdDnwdPos_Val : Constant  Value=KeSMSwAcsMd8SecRwLtStBkReclnUpwdDnwdPos_Val
  PA_KeSMSwRecoveryMdSecRwLtStBkReclnUpwdDnwdPosMax_Val : Constant  Value=KeSMSwRecoveryMdSecRwLtStBkReclnUpwdDnwdPosMax_Val
  PA_KeSMSwRecoveryMdSecRwLtStBkReclnUpwdDnwdPosMin_Val : Constant  Value=KeSMSwRecoveryMdSecRwLtStBkReclnUpwdDnwdPosMin_Val
  PA_KeSMSwRecoveryMdSecRwLtStBkReclnUpwdDnwdPos_Val : Constant  Value=KeSMSwRecoveryMdSecRwLtStBkReclnUpwdDnwdPos_Val
  PA_KeSMSwVIPSecRwLtStBkReclnUpwdDnwdPosMax_Val : Constant  Value=KeSMSwVIPSecRwLtStBkReclnUpwdDnwdPosMax_Val
  PA_KeSMSwVIPSecRwLtStBkReclnUpwdDnwdPosMin_Val : Constant  Value=KeSMSwVIPSecRwLtStBkReclnUpwdDnwdPosMin_Val
  PA_KeSMSwVIPSecRwLtStBkReclnUpwdDnwdPos_Val : Constant  Value=KeSMSwVIPSecRwLtStBkReclnUpwdDnwdPos_Val
  Terminator_{1..63} (63 alike) : Terminator
  wires:
  PA_KeSMSw4SAcsMd21SecRwLtStBkReclnUpwdDnwdPosMax_Val/1 -> Terminator_1/1
  PA_KeSMSw4SAcsMd21SecRwLtStBkReclnUpwdDnwdPosMin_Val/1 -> Terminator_2/1
  PA_KeSMSw4SAcsMd21SecRwLtStBkReclnUpwdDnwdPos_Val/1 -> Terminator_3/1
  PA_KeSMSw4SAcsMd22SecRwLtStBkReclnUpwdDnwdPos1Max_Val/1 -> Terminator_4/1
  PA_KeSMSw4SAcsMd22SecRwLtStBkReclnUpwdDnwdPos1Min_Val/1 -> Terminator_5/1
  PA_KeSMSw4SAcsMd22SecRwLtStBkReclnUpwdDnwdPos1_Val/1 -> Terminator_6/1
  PA_KeSMSw4SAcsMd22SecRwLtStBkReclnUpwdDnwdPos2Max_Val/1 -> Terminator_7/1
  PA_KeSMSw4SAcsMd22SecRwLtStBkReclnUpwdDnwdPos2Min_Val/1 -> Terminator_8/1
  PA_KeSMSw4SAcsMd22SecRwLtStBkReclnUpwdDnwdPos2_Val/1 -> Terminator_9/1
  PA_KeSMSw4SAcsMd25SecRwLtStBkReclnUpwdDnwdPosMax_Val/1 -> Terminator_10/1
  PA_KeSMSw4SAcsMd25SecRwLtStBkReclnUpwdDnwdPosMin_Val/1 -> Terminator_11/1
  PA_KeSMSw4SAcsMd25SecRwLtStBkReclnUpwdDnwdPos_Val/1 -> Terminator_12/1
  PA_KeSMSw4SAcsMd26SecRwLtStBkReclnUpwdDnwdPosMax_Val/1 -> Terminator_13/1
  PA_KeSMSw4SAcsMd26SecRwLtStBkReclnUpwdDnwdPosMin_Val/1 -> Terminator_14/1
  PA_KeSMSw4SAcsMd26SecRwLtStBkReclnUpwdDnwdPos_Val/1 -> Terminator_15/1
  PA_KeSMSw4sLyingMDSecRwLtStBkReclnUpwdDnwdPosMax_Val/1 -> Terminator_16/1
  PA_KeSMSw4sLyingMDSecRwLtStBkReclnUpwdDnwdPosMin_Val/1 -> Terminator_17/1
  PA_KeSMSw4sLyingMDSecRwLtStBkReclnUpwdDnwdPos_Val/1 -> Terminator_18/1
  PA_KeSMSw4sRecoveryMDSecRwLtStBkReclnUpwdDnwdPosMax_Val/1 -> Terminator_19/1
  PA_KeSMSw4sRecoveryMDSecRwLtStBkReclnUpwdDnwdPosMin_Val/1 -> Terminator_20/1
  PA_KeSMSw4sRecoveryMDSecRwLtStBkReclnUpwdDnwdPos_Val/1 -> Terminator_21/1
  PA_KeSMSw4sVIPMDSecRwLtStBkReclnUpwdDnwdPosMax_Val/1 -> Terminator_22/1
  PA_KeSMSw4sVIPMDSecRwLtStBkReclnUpwdDnwdPosMin_Val/1 -> Terminator_23/1
  PA_KeSMSw4sVIPMDSecRwLtStBkReclnUpwdDnwdPos_Val/1 -> Terminator_24/1
  PA_KeSMSw6sAcsEntrySecRwLtStBkReclnUpwdDnwd1Pos_Val/1 -> Terminator_25/1
  PA_KeSMSw6sAcsEntrySecRwLtStBkReclnUpwdDnwdPos1Max_Val/1 -> Terminator_26/1
  PA_KeSMSw6sAcsEntrySecRwLtStBkReclnUpwdDnwdPos1Min_Val/1 -> Terminator_27/1
  PA_KeSMSw6sAcsEntrySecRwLtStBkReclnUpwdDnwdPosMax_Val/1 -> Terminator_28/1
  PA_KeSMSw6sAcsEntrySecRwLtStBkReclnUpwdDnwdPosMin_Val/1 -> Terminator_29/1
  PA_KeSMSw6sAcsEntrySecRwLtStBkReclnUpwdDnwdPos_Val/1 -> Terminator_30/1
  PA_KeSMSw6sAcsExtSecRwLtStBkReclnUpwdDnwdPosMax_Val/1 -> Terminator_31/1
  PA_KeSMSw6sAcsExtSecRwLtStBkReclnUpwdDnwdPosMin_Val/1 -> Terminator_32/1
  PA_KeSMSw6sAcsExtSecRwLtStBkReclnUpwdDnwdPos_Val/1 -> Terminator_33/1
  PA_KeSMSw6sRecoveryMdSecRwLtStBkReclnUpwdDnwdPosMax_Val/1 -> Terminator_34/1
  PA_KeSMSw6sRecoveryMdSecRwLtStBkReclnUpwdDnwdPosMin_Val/1 -> Terminator_35/1
  PA_KeSMSw6sRecoveryMdSecRwLtStBkReclnUpwdDnwdPos_Val/1 -> Terminator_36/1
  PA_KeSMSw6sVIPSecRwLtStBkReclnUpwdDnwdPosMax_Val/1 -> Terminator_37/1
  PA_KeSMSw6sVIPSecRwLtStBkReclnUpwdDnwdPosMin_Val/1 -> Terminator_38/1
  PA_KeSMSw6sVIPSecRwLtStBkReclnUpwdDnwdPos_Val/1 -> Terminator_39/1
  PA_KeSMSwAcsEntrySecRwLtStBkReclnUpwdDnwdPos1Max_Val/1 -> Terminator_40/1
  PA_KeSMSwAcsEntrySecRwLtStBkReclnUpwdDnwdPos1Min_Val/1 -> Terminator_41/1
  PA_KeSMSwAcsEntrySecRwLtStBkReclnUpwdDnwdPos1_Val/1 -> Terminator_42/1
  PA_KeSMSwAcsEntrySecRwLtStBkReclnUpwdDnwdPosMax_Val/1 -> Terminator_43/1
  PA_KeSMSwAcsEntrySecRwLtStBkReclnUpwdDnwdPosMin_Val/1 -> Terminator_44/1
  PA_KeSMSwAcsEntrySecRwLtStBkReclnUpwdDnwdPos_Val/1 -> Terminator_45/1
  PA_KeSMSwAcsExtSecRwLtStBkReclnUpwdDnwdPosMax_Val/1 -> Terminator_46/1
  PA_KeSMSwAcsExtSecRwLtStBkReclnUpwdDnwdPosMin_Val/1 -> Terminator_47/1
  PA_KeSMSwAcsExtSecRwLtStBkReclnUpwdDnwdPos_Val/1 -> Terminator_48/1
  PA_KeSMSwRecoveryMdSecRwLtStBkReclnUpwdDnwdPosMax_Val/1 -> Terminator_49/1
  PA_KeSMSwRecoveryMdSecRwLtStBkReclnUpwdDnwdPosMin_Val/1 -> Terminator_50/1
  PA_KeSMSwRecoveryMdSecRwLtStBkReclnUpwdDnwdPos_Val/1 -> Terminator_51/1
  PA_KeSMSwVIPSecRwLtStBkReclnUpwdDnwdPosMax_Val/1 -> Terminator_52/1
  PA_KeSMSwVIPSecRwLtStBkReclnUpwdDnwdPosMin_Val/1 -> Terminator_53/1
  PA_KeSMSwVIPSecRwLtStBkReclnUpwdDnwdPos_Val/1 -> Terminator_54/1
  PA_KeSMSwAcsMd32SecRwLtStBkReclnUpwdDnwdPos1Max_Val/1 -> Terminator_55/1
  PA_KeSMSwAcsMd32SecRwLtStBkReclnUpwdDnwdPos1Min_Val/1 -> Terminator_56/1
  PA_KeSMSwAcsMd32SecRwLtStBkReclnUpwdDnwdPos1_Val/1 -> Terminator_57/1
  PA_KeSMSwAcsMd32SecRwLtStBkReclnUpwdDnwdPosMax_Val/1 -> Terminator_58/1
  PA_KeSMSwAcsMd32SecRwLtStBkReclnUpwdDnwdPosMin_Val/1 -> Terminator_59/1
  PA_KeSMSwAcsMd32SecRwLtStBkReclnUpwdDnwdPos_Val/1 -> Terminator_60/1
  PA_KeSMSwAcsMd8SecRwLtStBkReclnUpwdDnwdPosMax_Val/1 -> Terminator_61/1
  PA_KeSMSwAcsMd8SecRwLtStBkReclnUpwdDnwdPosMin_Val/1 -> Terminator_62/1
  PA_KeSMSwAcsMd8SecRwLtStBkReclnUpwdDnwdPos_Val/1 -> Terminator_63/1

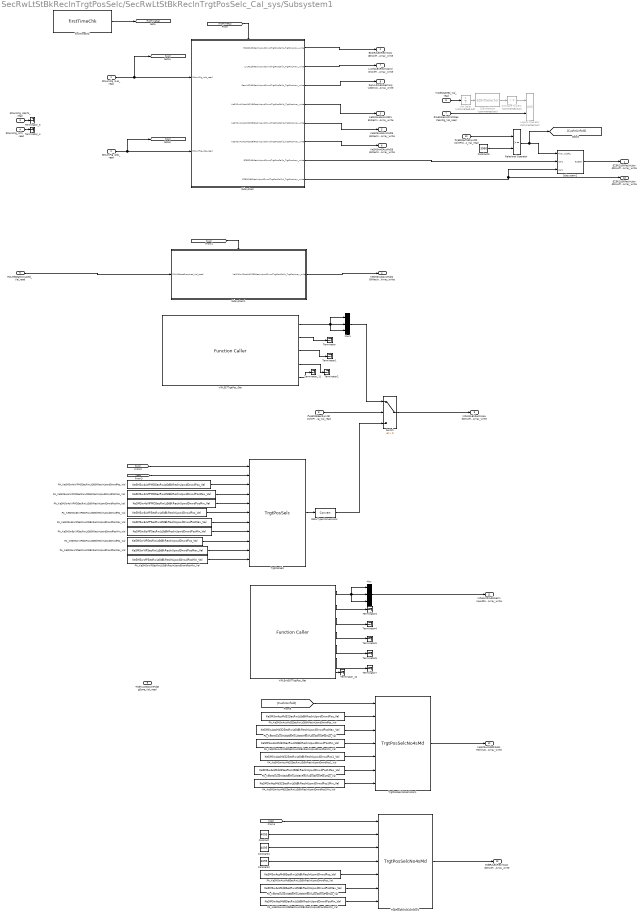
== system SecRwLtStBkReclnTrgtPosSelc/SecRwLtStBkReclnTrgtPosSelc_Cal_sys/Subsystem1 ==
  StNumFlg_Is4s_read : Inport
  StNumFlg_Is6s_read : Inport  Port=2
  StNumFlg_Is6s7s_read : Inport  Port=3
  StNumFlg_Is7s_read : Inport  Port=4
  R2LMdSeatOccupied_Val_read : Inport  Port=5
  modestate32_Val_read : Inport  Port=6
  R2LBkReclinFirstStepPassFlg_Val_read : Inport  Port=7
  IfVeSMSbSecRwLtStCshnFrntUpwdDnwdMovConfig_Val_read : Inport  Port=8
  ThdRwLtStCshnFldStgDone_Val_read : Inport  Port=9
  IfVeSMSuThdRwLtStCshnFldUpwdDnwdPos_Val_read : Inport  Port=10
  32BitSelector : StIsPosChkLib/32BitSelector  Commented=on  BitNum=0
  Compare To Zero : simulink/Logic and Bit Operations/Compare To Zero  Commented=on  relop=>  OutDataTypeStr=boolean
  Constant : Constant  Value=4095  OutDataTypeStr=uint16
  Constant1 : Constant  Value=4095  OutDataTypeStr=uint16
  Constant2 : Constant  Value=4095  OutDataTypeStr=uint16
  Constant3 : Constant  Value=3960  OutDataTypeStr=uint16
  Data Type Conversion4 : DataTypeConversion
  Logical Operator : Logic  Commented=on  AllPortsSameDT=off  OutDataTypeStr=boolean
  Mux : Mux  Inputs=3
  Mux1 : Mux  Inputs=3
  PA_KeSMSw4sVIPMDSecRwLtStBkReclnUpwdDnwdPosMax_Val : Constant  Value=KeSMSw4sVIPMDSecRwLtStBkReclnUpwdDnwdPosMax_Val
  PA_KeSMSw4sVIPMDSecRwLtStBkReclnUpwdDnwdPosMin_Val : Constant  Value=KeSMSw4sVIPMDSecRwLtStBkReclnUpwdDnwdPosMin_Val
  PA_KeSMSw4sVIPMDSecRwLtStBkReclnUpwdDnwdPos_Val : Constant  Value=KeSMSw4sVIPMDSecRwLtStBkReclnUpwdDnwdPos_Val
  PA_KeSMSw6sVIPSecRwLtStBkReclnUpwdDnwdPosMax_Val : Constant  Value=KeSMSw6sVIPSecRwLtStBkReclnUpwdDnwdPosMax_Val
  PA_KeSMSw6sVIPSecRwLtStBkReclnUpwdDnwdPosMin_Val : Constant  Value=KeSMSw6sVIPSecRwLtStBkReclnUpwdDnwdPosMin_Val
  PA_KeSMSw6sVIPSecRwLtStBkReclnUpwdDnwdPos_Val : Constant  Value=KeSMSw6sVIPSecRwLtStBkReclnUpwdDnwdPos_Val
  PA_KeSMSwAcsMd32SecRwLtStBkReclnUpwdDnwdPos1Max_Val : Constant  Value=KeSMSwAcsMd32SecRwLtStBkReclnUpwdDnwdPos1Max_Val
  PA_KeSMSwAcsMd32SecRwLtStBkReclnUpwdDnwdPos1Min_Val : Constant  Value=KeSMSwAcsMd32SecRwLtStBkReclnUpwdDnwdPos1Min_Val
  PA_KeSMSwAcsMd32SecRwLtStBkReclnUpwdDnwdPos1_Val : Constant  Value=KeSMSwAcsMd32SecRwLtStBkReclnUpwdDnwdPos1_Val
  PA_KeSMSwAcsMd32SecRwLtStBkReclnUpwdDnwdPosMax_Val : Constant  Value=KeSMSwAcsMd32SecRwLtStBkReclnUpwdDnwdPosMax_Val
  PA_KeSMSwAcsMd32SecRwLtStBkReclnUpwdDnwdPosMin_Val : Constant  Value=KeSMSwAcsMd32SecRwLtStBkReclnUpwdDnwdPosMin_Val
  PA_KeSMSwAcsMd32SecRwLtStBkReclnUpwdDnwdPos_Val : Constant  Value=KeSMSwAcsMd32SecRwLtStBkReclnUpwdDnwdPos_Val
  PA_KeSMSwAcsMd8SecRwLtStBkReclnUpwdDnwdPosMax_Val : Constant  Value=KeSMSwAcsMd8SecRwLtStBkReclnUpwdDnwdPosMax_Val
  PA_KeSMSwAcsMd8SecRwLtStBkReclnUpwdDnwdPosMin_Val : Constant  Value=KeSMSwAcsMd8SecRwLtStBkReclnUpwdDnwdPosMin_Val
  PA_KeSMSwAcsMd8SecRwLtStBkReclnUpwdDnwdPos_Val : Constant  Value=KeSMSwAcsMd8SecRwLtStBkReclnUpwdDnwdPos_Val
  PA_KeSMSwVIPSecRwLtStBkReclnUpwdDnwdPosMax_Val : Constant  Value=KeSMSwVIPSecRwLtStBkReclnUpwdDnwdPosMax_Val
  PA_KeSMSwVIPSecRwLtStBkReclnUpwdDnwdPosMin_Val : Constant  Value=KeSMSwVIPSecRwLtStBkReclnUpwdDnwdPosMin_Val
  PA_KeSMSwVIPSecRwLtStBkReclnUpwdDnwdPos_Val : Constant  Value=KeSMSwVIPSecRwLtStBkReclnUpwdDnwdPos_Val
  Relational Operator : RelationalOperator  OutDataTypeStr=boolean  RndMeth=Simplest
  Subsystem : Subsystem
  Subsystem1 : Subsystem
  Subsystem2 : Subsystem
  Switch : Switch  Criteria=u2 > Threshold
  Terminator{,1..7} (8 alike) : Terminator
  Terminator_{3..4,11..12} (4 alike) : Terminator
  TrgtPosSelc : TrgtPosSelcLib/TrgtPosSelc  SystemSampleTime=-1
  TrgtPosSelcNot4sMotor1 : TrgtPosSelcLib/TrgtPosSelcNo4sMd  SystemSampleTime=-1
  TrgtPosSelcNot4sMotor2 : TrgtPosSelcLib/TrgtPosSelcNo4sMd  SystemSampleTime=-1
  Unit Delay : UnitDelay  Commented=on  SampleTime=-1
  VIPL557TrgtPos_Get : FunctionCaller  FunctionPrototype=[SecRwLtStBkReclnTrgtPos,SecRwLtStZeroTrgtPos,SecRwLtStLgrstUpwdDnwdTrgtPos,SecRwLtStLgrstInwdOtwdTrgtPos,SecRwLtStFwdBkwdTrgtPos] = VIPL557TrgtPos_Get()  OutputArgumentSpecifications=uint16(1), uint16(1), uint16(1), uint16(1), uint16(1)
  VIPLExit557TrgtPos_Get : FunctionCaller  FunctionPrototype=[SecRwLtStBkReclnTrgtPos,SecRwLtStZeroTrgtPos,SecRwLtStLgrstUpwdDnwdTrgtPos,SecRwLtStLgrstInwdOtwdTrgtPos,ThdRwLtStBkReclnTrgtPos,ThdRwLtStFwdBkwdTrgtPos,SecRwLtStFwdBkwdTrgtPos] = VIPLExit557TrgtPos_Get()  OutputArgumentSpecifications=uint16(1), uint16(1), uint16(1), uint16(1), uint16(1), uint16(1), uint16(1)
  firstTimeChk : TrgtPosSelcLib/firstTimeChk  SystemSampleTime=-1
  EZER2LBkReclnUpwdDnwdTrgtPosCalib_TrgtPosArray_write : Outport
      settings: EnsureOutportIsVirtual=on
  EZQR2LBkReclnUpwdDnwdTrgtPosCalib_TrgtPosArray_write : Outport  Port=2
      settings: EnsureOutportIsVirtual=on
  KeSMSw4SAcsMd21BkReclnUpwdDnwdTrgtPosCalib_TrgtPosArray_write : Outport  Port=3
      settings: EnsureOutportIsVirtual=on
  KeSMSw4SAcsMd22BkReclnUpwdDnwdTrgtPosCalib_TrgtPosArray_write : Outport  Port=4
      settings: EnsureOutportIsVirtual=on
  KeSMSw4SAcsMd25BkReclnUpwdDnwdTrgtPosCalib_TrgtPosArray_write : Outport  Port=5
      settings: EnsureOutportIsVirtual=on
  KeSMSw4SAcsMd26BkReclnUpwdDnwdTrgtPosCalib_TrgtPosArray_write : Outport  Port=6
      settings: EnsureOutportIsVirtual=on
  LyLR2LBkReclnUpwdDnwdTrgtPosCalib_TrgtPosArray_write : Outport  Port=7
      settings: EnsureOutportIsVirtual=on
  RecvLR2LBkReclnUpwdDnwdTrgtPosCalib_TrgtPosArray_write : Outport  Port=8
      settings: EnsureOutportIsVirtual=on
  VIPLR2LBkReclnUpwdDnwdTrgtPosCalib_TrgtPosArray_write : Outport  Port=9
      settings: EnsureOutportIsVirtual=on
  EZER2LBkReclnUpwdDnwdTrgtPosCalib1_TrgtPosArray_write : Outport  Port=10
      settings: EnsureOutportIsVirtual=on
  VIPLExitR2LBkReclnUpwdDnwdTrgtPosCalib_TrgtPosArray_write : Outport  Port=11
      settings: EnsureOutportIsVirtual=on
  KeSMSwMd32R2LBkReclnUpwdDnwdTrgtPosCalib_TrgtPosArray_write : Outport  Port=12
      settings: EnsureOutportIsVirtual=on
  Md8R2LBkReclnUpwdDnwdTrgtPosCalib_TrgtPosArray_write : Outport  Port=13
      settings: EnsureOutportIsVirtual=on
  wires:
  StNumFlg_Is4s_read/1 -> [is4s], Subsystem/1(StNumFlg_Is4s_read)
  StNumFlg_Is7s_read/1 -> Terminator_4/1
  Subsystem/2(LyLR2LBkReclnUpwdDnwdTrgtPosCalib_TrgtPosArray_write) -> LyLR2LBkReclnUpwdDnwdTrgtPosCalib_TrgtPosArray_write/1
  Subsystem/1(EZQR2LBkReclnUpwdDnwdTrgtPosCalib_TrgtPosArray_write) -> EZQR2LBkReclnUpwdDnwdTrgtPosCalib_TrgtPosArray_write/1
  firstTimeChk/1 -> [firstTimeflg]
  Switch/1 -> VIPLR2LBkReclnUpwdDnwdTrgtPosCalib_TrgtPosArray_write/1
  StNumFlg_Is6s7s_read/1 -> Terminator_3/1
  [firstTimeflg] -> Subsystem/Enable
  StNumFlg_Is6s_read/1 -> [is6s], Subsystem/2(StNumFlg_Is6s_read)
  Subsystem/3(RecvLR2LBkReclnUpwdDnwdTrgtPosCalib_TrgtPosArray_write) -> RecvLR2LBkReclnUpwdDnwdTrgtPosCalib_TrgtPosArray_write/1
  Subsystem/4(KeSMSw4SAcsMd21BkReclnUpwdDnwdTrgtPosCalib_TrgtPosArray_write) -> KeSMSw4SAcsMd21BkReclnUpwdDnwdTrgtPosCalib_TrgtPosArray_write/1
  Subsystem/5(KeSMSw4SAcsMd25BkReclnUpwdDnwdTrgtPosCalib_TrgtPosArray_write) -> KeSMSw4SAcsMd25BkReclnUpwdDnwdTrgtPosCalib_TrgtPosArray_write/1
  Subsystem/6(KeSMSw4SAcsMd26BkReclnUpwdDnwdTrgtPosCalib_TrgtPosArray_write) -> KeSMSw4SAcsMd26BkReclnUpwdDnwdTrgtPosCalib_TrgtPosArray_write/1
  R2LMdSeatOccupied_Val_read/1 -> Subsystem1/1(R2LMdSeatOccupied_Val_read)
  Subsystem1/1(KeSMSw4SAcsMd22BkReclnUpwdDnwdTrgtPosCalib_TrgtPosArray_write) -> KeSMSw4SAcsMd22BkReclnUpwdDnwdTrgtPosCalib_TrgtPosArray_write/1
  [is4s] -> Subsystem1/Enable
  Subsystem/8(EZER2LBkReclnUpwdDnwdTrgtPosCalib1_TrgtPosArray_write) -> Subsystem2/3(Cal1), EZER2LBkReclnUpwdDnwdTrgtPosCalib1_TrgtPosArray_write/1
  Subsystem/7(EZER2LBkReclnUpwdDnwdTrgtPosCalib_TrgtPosArray_write) -> Subsystem2/2(Cal2)
  Subsystem2/1(EZECal) -> EZER2LBkReclnUpwdDnwdTrgtPosCalib_TrgtPosArray_write/1
  modestate32_Val_read/1 -> Unit Delay/1
  R2LBkReclinFirstStepPassFlg_Val_read/1 -> Logical Operator/2
  Unit Delay/1 -> 32BitSelector/1
  32BitSelector/1 -> Compare To Zero/1
  Compare To Zero/1 -> Logical Operator/1
  PA_KeSMSw6sVIPSecRwLtStBkReclnUpwdDnwdPosMax_Val/1 -> TrgtPosSelc/7
  PA_KeSMSwVIPSecRwLtStBkReclnUpwdDnwdPosMax_Val/1 -> TrgtPosSelc/10
  PA_KeSMSw4sVIPMDSecRwLtStBkReclnUpwdDnwdPos_Val/1 -> TrgtPosSelc/3
  PA_KeSMSw4sVIPMDSecRwLtStBkReclnUpwdDnwdPosMax_Val/1 -> TrgtPosSelc/4
  TrgtPosSelc/1 -> Data Type Conversion4/1
  [is6s] -> TrgtPosSelc/2
  PA_KeSMSw6sVIPSecRwLtStBkReclnUpwdDnwdPos_Val/1 -> TrgtPosSelc/6
  PA_KeSMSw4sVIPMDSecRwLtStBkReclnUpwdDnwdPosMin_Val/1 -> TrgtPosSelc/5
  PA_KeSMSwVIPSecRwLtStBkReclnUpwdDnwdPosMin_Val/1 -> TrgtPosSelc/11
  [is4s] -> TrgtPosSelc/1
  PA_KeSMSw6sVIPSecRwLtStBkReclnUpwdDnwdPosMin_Val/1 -> TrgtPosSelc/8
  PA_KeSMSwVIPSecRwLtStBkReclnUpwdDnwdPos_Val/1 -> TrgtPosSelc/9
  Mux1/1 -> Switch/1
  VIPL557TrgtPos_Get/1 -> Mux1/3, Mux1/2, Mux1/1
  IfVeSMSbSecRwLtStCshnFrntUpwdDnwdMovConfig_Val_read/1 -> Switch/2
  Data Type Conversion4/1 -> Switch/3
  VIPL557TrgtPos_Get/2 -> Terminator/1
  VIPL557TrgtPos_Get/3 -> Terminator1/1
  VIPL557TrgtPos_Get/4 -> Terminator2/1
  Mux/1 -> VIPLExitR2LBkReclnUpwdDnwdTrgtPosCalib_TrgtPosArray_write/1
  VIPLExit557TrgtPos_Get/1 -> Mux/3, Mux/1, Mux/2
  VIPLExit557TrgtPos_Get/2 -> Terminator3/1
  VIPLExit557TrgtPos_Get/4 -> Terminator5/1
  VIPLExit557TrgtPos_Get/3 -> Terminator4/1
  VIPLExit557TrgtPos_Get/5 -> Terminator6/1
  VIPLExit557TrgtPos_Get/6 -> Terminator7/1
  VIPL557TrgtPos_Get/5 -> Terminator_11/1
  VIPLExit557TrgtPos_Get/7 -> Terminator_12/1
  PA_KeSMSwAcsMd32SecRwLtStBkReclnUpwdDnwdPos_Val/1 -> TrgtPosSelcNot4sMotor1/2
  PA_KeSMSwAcsMd32SecRwLtStBkReclnUpwdDnwdPosMax_Val/1 -> TrgtPosSelcNot4sMotor1/3
  PA_KeSMSwAcsMd32SecRwLtStBkReclnUpwdDnwdPosMin_Val/1 -> TrgtPosSelcNot4sMotor1/4
  PA_KeSMSwAcsMd32SecRwLtStBkReclnUpwdDnwdPos1_Val/1 -> TrgtPosSelcNot4sMotor1/5
  PA_KeSMSwAcsMd32SecRwLtStBkReclnUpwdDnwdPos1Max_Val/1 -> TrgtPosSelcNot4sMotor1/6
  PA_KeSMSwAcsMd32SecRwLtStBkReclnUpwdDnwdPos1Min_Val/1 -> TrgtPosSelcNot4sMotor1/7
  TrgtPosSelcNot4sMotor1/1 -> KeSMSwMd32R2LBkReclnUpwdDnwdTrgtPosCalib_TrgtPosArray_write/1
  [is6s] -> TrgtPosSelcNot4sMotor2/1
  PA_KeSMSwAcsMd8SecRwLtStBkReclnUpwdDnwdPosMin_Val/1 -> TrgtPosSelcNot4sMotor2/7
  PA_KeSMSwAcsMd8SecRwLtStBkReclnUpwdDnwdPosMax_Val/1 -> TrgtPosSelcNot4sMotor2/6
  PA_KeSMSwAcsMd8SecRwLtStBkReclnUpwdDnwdPos_Val/1 -> TrgtPosSelcNot4sMotor2/5
  Constant2/1 -> TrgtPosSelcNot4sMotor2/4
  Constant1/1 -> TrgtPosSelcNot4sMotor2/3
  Constant/1 -> TrgtPosSelcNot4sMotor2/2
  TrgtPosSelcNot4sMotor2/1 -> Md8R2LBkReclnUpwdDnwdTrgtPosCalib_TrgtPosArray_write/1
  IfVeSMSuThdRwLtStCshnFldUpwdDnwdPos_Val_read/1 -> Relational Operator/1
  Constant3/1 -> Relational Operator/2
  Relational Operator/1 -> [CushnUnfold], Subsystem2/1(FirstStepPassFlg)
  [CushnUnfold] -> TrgtPosSelcNot4sMotor1/1
